simulink model "ADU_Integration_R2014a_simulation"  (R2014a)
settings: Solver=FixedStepDiscrete  StartTime=285  StopTime=300  FixedStep=0.01  RelTol=1e-3
PostLoadFcn:
  | , if any(exist('dsrtsu_mdlpostloadfcn', 'file') == [2, 3, 6]), try dsrtsu_mdlpostloadfcn('Execute', bdroot); catch fprintf('Error in PostLoadFcn (dsrtsu_mdlpostloadfcn) for model "%s":\n %s\n', bdroot, lasterr); end, end,
InitFcn:
  | load 'data/chi2_dat';
  | load 'data/Line_struct';
  | load 'data/innerLNM_1';
  | load 'data/middleLNM_2';
  | load 'data/outerLNM_1';
  | load 'data/landmarks_patac_schimmel_ccw';
  | load 'data/patac_navi_array';
  | load 'data/sensor';
  | load 'data/map_struct';
  | addpath map_src
  | Integration_Parameter;
  | load 'TestData_001';
values from neighbouring files (symbols this model uses):
  TestData_001 =     [TestData_001.mat]
undefined symbols (not defined in the file or in its folder): chi2_dat, innerLNM_1, landmarks_patac_schimmel_ccw, middleLNM_2, outerLNM_1, patac_navi_array
libraries: simulink x36, rtican x1
(part 6 of 22)

== system ADU_Integration_R2014a_simulation/LogData/Sensor_ESR/Data_51 ==
  1-D Lookup Table1 : Lookup_n-D  NumberOfTableDimensions=1  BreakpointsForDimension1=TestData_001.X.Data  Table=TestData_001.Y(206+4*a).Data  RndMeth=Simplest  InputSameDT=on
  1-D Lookup Table2 : Lookup_n-D  NumberOfTableDimensions=1  BreakpointsForDimension1=TestData_001.X.Data  Table=TestData_001.Y(205+4*a).Data  RndMeth=Simplest  InputSameDT=on
  1-D Lookup Table3 : Lookup_n-D  NumberOfTableDimensions=1  BreakpointsForDimension1=TestData_001.X.Data  Table=TestData_001.Y(207+4*a).Data  RndMeth=Simplest  InputSameDT=on
  1-D Lookup Table4 : Lookup_n-D  NumberOfTableDimensions=1  BreakpointsForDimension1=TestData_001.X.Data  Table=TestData_001.Y(208+4*a).Data  RndMeth=Simplest  InputSameDT=on
  Mux5 : Mux
  Quantizer9 : Quantizer  QuantizationInterval=1
  Out1 : Outport
  wires:
  Mux5/1 -> Out1/1
  [Clock] -> 1-D Lookup Table2/1, 1-D Lookup Table4/1, 1-D Lookup Table3/1, 1-D Lookup Table1/1
  1-D Lookup Table4/1 -> Mux5/4
  Quantizer9/1 -> Mux5/1
  1-D Lookup Table2/1 -> Quantizer9/1
  1-D Lookup Table1/1 -> Mux5/2  "Data"
  1-D Lookup Table3/1 -> Mux5/3

== system ADU_Integration_R2014a_simulation/LogData/Sensor_ESR/Data_52 ==
  1-D Lookup Table1 : Lookup_n-D  NumberOfTableDimensions=1  BreakpointsForDimension1=TestData_001.X.Data  Table=TestData_001.Y(206+4*a).Data  RndMeth=Simplest  InputSameDT=on
  1-D Lookup Table2 : Lookup_n-D  NumberOfTableDimensions=1  BreakpointsForDimension1=TestData_001.X.Data  Table=TestData_001.Y(205+4*a).Data  RndMeth=Simplest  InputSameDT=on
  1-D Lookup Table3 : Lookup_n-D  NumberOfTableDimensions=1  BreakpointsForDimension1=TestData_001.X.Data  Table=TestData_001.Y(207+4*a).Data  RndMeth=Simplest  InputSameDT=on
  1-D Lookup Table4 : Lookup_n-D  NumberOfTableDimensions=1  BreakpointsForDimension1=TestData_001.X.Data  Table=TestData_001.Y(208+4*a).Data  RndMeth=Simplest  InputSameDT=on
  Mux5 : Mux
  Quantizer9 : Quantizer  QuantizationInterval=1
  Out1 : Outport
  wires:
  1-D Lookup Table3/1 -> Mux5/3
  1-D Lookup Table1/1 -> Mux5/2  "Data"
  1-D Lookup Table2/1 -> Quantizer9/1
  Quantizer9/1 -> Mux5/1
  1-D Lookup Table4/1 -> Mux5/4
  [Clock] -> 1-D Lookup Table1/1, 1-D Lookup Table3/1, 1-D Lookup Table4/1, 1-D Lookup Table2/1
  Mux5/1 -> Out1/1

== system ADU_Integration_R2014a_simulation/LogData/Sensor_ESR/Data_53 ==
  1-D Lookup Table1 : Lookup_n-D  NumberOfTableDimensions=1  BreakpointsForDimension1=TestData_001.X.Data  Table=TestData_001.Y(206+4*a).Data  RndMeth=Simplest  InputSameDT=on
  1-D Lookup Table2 : Lookup_n-D  NumberOfTableDimensions=1  BreakpointsForDimension1=TestData_001.X.Data  Table=TestData_001.Y(205+4*a).Data  RndMeth=Simplest  InputSameDT=on
  1-D Lookup Table3 : Lookup_n-D  NumberOfTableDimensions=1  BreakpointsForDimension1=TestData_001.X.Data  Table=TestData_001.Y(207+4*a).Data  RndMeth=Simplest  InputSameDT=on
  1-D Lookup Table4 : Lookup_n-D  NumberOfTableDimensions=1  BreakpointsForDimension1=TestData_001.X.Data  Table=TestData_001.Y(208+4*a).Data  RndMeth=Simplest  InputSameDT=on
  Mux5 : Mux
  Quantizer9 : Quantizer  QuantizationInterval=1
  Out1 : Outport
  wires:
  Mux5/1 -> Out1/1
  [Clock] -> 1-D Lookup Table2/1, 1-D Lookup Table4/1, 1-D Lookup Table3/1, 1-D Lookup Table1/1
  1-D Lookup Table4/1 -> Mux5/4
  Quantizer9/1 -> Mux5/1
  1-D Lookup Table2/1 -> Quantizer9/1
  1-D Lookup Table1/1 -> Mux5/2  "Data"
  1-D Lookup Table3/1 -> Mux5/3

== system ADU_Integration_R2014a_simulation/LogData/Sensor_ESR/Data_54 ==
  1-D Lookup Table1 : Lookup_n-D  NumberOfTableDimensions=1  BreakpointsForDimension1=TestData_001.X.Data  Table=TestData_001.Y(206+4*a).Data  RndMeth=Simplest  InputSameDT=on
  1-D Lookup Table2 : Lookup_n-D  NumberOfTableDimensions=1  BreakpointsForDimension1=TestData_001.X.Data  Table=TestData_001.Y(205+4*a).Data  RndMeth=Simplest  InputSameDT=on
  1-D Lookup Table3 : Lookup_n-D  NumberOfTableDimensions=1  BreakpointsForDimension1=TestData_001.X.Data  Table=TestData_001.Y(207+4*a).Data  RndMeth=Simplest  InputSameDT=on
  1-D Lookup Table4 : Lookup_n-D  NumberOfTableDimensions=1  BreakpointsForDimension1=TestData_001.X.Data  Table=TestData_001.Y(208+4*a).Data  RndMeth=Simplest  InputSameDT=on
  Mux5 : Mux
  Quantizer9 : Quantizer  QuantizationInterval=1
  Out1 : Outport
  wires:
  1-D Lookup Table3/1 -> Mux5/3
  1-D Lookup Table1/1 -> Mux5/2  "Data"
  1-D Lookup Table2/1 -> Quantizer9/1
  Quantizer9/1 -> Mux5/1
  1-D Lookup Table4/1 -> Mux5/4
  [Clock] -> 1-D Lookup Table1/1, 1-D Lookup Table3/1, 1-D Lookup Table4/1, 1-D Lookup Table2/1
  Mux5/1 -> Out1/1

== system ADU_Integration_R2014a_simulation/LogData/Sensor_ESR/Data_55 ==
  1-D Lookup Table1 : Lookup_n-D  NumberOfTableDimensions=1  BreakpointsForDimension1=TestData_001.X.Data  Table=TestData_001.Y(206+4*a).Data  RndMeth=Simplest  InputSameDT=on
  1-D Lookup Table2 : Lookup_n-D  NumberOfTableDimensions=1  BreakpointsForDimension1=TestData_001.X.Data  Table=TestData_001.Y(205+4*a).Data  RndMeth=Simplest  InputSameDT=on
  1-D Lookup Table3 : Lookup_n-D  NumberOfTableDimensions=1  BreakpointsForDimension1=TestData_001.X.Data  Table=TestData_001.Y(207+4*a).Data  RndMeth=Simplest  InputSameDT=on
  1-D Lookup Table4 : Lookup_n-D  NumberOfTableDimensions=1  BreakpointsForDimension1=TestData_001.X.Data  Table=TestData_001.Y(208+4*a).Data  RndMeth=Simplest  InputSameDT=on
  Mux5 : Mux
  Quantizer9 : Quantizer  QuantizationInterval=1
  Out1 : Outport
  wires:
  Mux5/1 -> Out1/1
  [Clock] -> 1-D Lookup Table2/1, 1-D Lookup Table4/1, 1-D Lookup Table3/1, 1-D Lookup Table1/1
  1-D Lookup Table4/1 -> Mux5/4
  Quantizer9/1 -> Mux5/1
  1-D Lookup Table2/1 -> Quantizer9/1
  1-D Lookup Table1/1 -> Mux5/2  "Data"
  1-D Lookup Table3/1 -> Mux5/3

== system ADU_Integration_R2014a_simulation/LogData/Sensor_ESR/Data_56 ==
  1-D Lookup Table1 : Lookup_n-D  NumberOfTableDimensions=1  BreakpointsForDimension1=TestData_001.X.Data  Table=TestData_001.Y(206+4*a).Data  RndMeth=Simplest  InputSameDT=on
  1-D Lookup Table2 : Lookup_n-D  NumberOfTableDimensions=1  BreakpointsForDimension1=TestData_001.X.Data  Table=TestData_001.Y(205+4*a).Data  RndMeth=Simplest  InputSameDT=on
  1-D Lookup Table3 : Lookup_n-D  NumberOfTableDimensions=1  BreakpointsForDimension1=TestData_001.X.Data  Table=TestData_001.Y(207+4*a).Data  RndMeth=Simplest  InputSameDT=on
  1-D Lookup Table4 : Lookup_n-D  NumberOfTableDimensions=1  BreakpointsForDimension1=TestData_001.X.Data  Table=TestData_001.Y(208+4*a).Data  RndMeth=Simplest  InputSameDT=on
  Mux5 : Mux
  Quantizer9 : Quantizer  QuantizationInterval=1
  Out1 : Outport
  wires:
  1-D Lookup Table3/1 -> Mux5/3
  1-D Lookup Table1/1 -> Mux5/2  "Data"
  1-D Lookup Table2/1 -> Quantizer9/1
  Quantizer9/1 -> Mux5/1
  1-D Lookup Table4/1 -> Mux5/4
  [Clock] -> 1-D Lookup Table1/1, 1-D Lookup Table3/1, 1-D Lookup Table4/1, 1-D Lookup Table2/1
  Mux5/1 -> Out1/1

== system ADU_Integration_R2014a_simulation/LogData/Sensor_ESR/Data_57 ==
  1-D Lookup Table1 : Lookup_n-D  NumberOfTableDimensions=1  BreakpointsForDimension1=TestData_001.X.Data  Table=TestData_001.Y(206+4*a).Data  RndMeth=Simplest  InputSameDT=on
  1-D Lookup Table2 : Lookup_n-D  NumberOfTableDimensions=1  BreakpointsForDimension1=TestData_001.X.Data  Table=TestData_001.Y(205+4*a).Data  RndMeth=Simplest  InputSameDT=on
  1-D Lookup Table3 : Lookup_n-D  NumberOfTableDimensions=1  BreakpointsForDimension1=TestData_001.X.Data  Table=TestData_001.Y(207+4*a).Data  RndMeth=Simplest  InputSameDT=on
  1-D Lookup Table4 : Lookup_n-D  NumberOfTableDimensions=1  BreakpointsForDimension1=TestData_001.X.Data  Table=TestData_001.Y(208+4*a).Data  RndMeth=Simplest  InputSameDT=on
  Mux5 : Mux
  Quantizer9 : Quantizer  QuantizationInterval=1
  Out1 : Outport
  wires:
  Mux5/1 -> Out1/1
  [Clock] -> 1-D Lookup Table2/1, 1-D Lookup Table4/1, 1-D Lookup Table3/1, 1-D Lookup Table1/1
  1-D Lookup Table4/1 -> Mux5/4
  Quantizer9/1 -> Mux5/1
  1-D Lookup Table2/1 -> Quantizer9/1
  1-D Lookup Table1/1 -> Mux5/2  "Data"
  1-D Lookup Table3/1 -> Mux5/3

== system ADU_Integration_R2014a_simulation/LogData/Sensor_ESR/Data_58 ==
  1-D Lookup Table1 : Lookup_n-D  NumberOfTableDimensions=1  BreakpointsForDimension1=TestData_001.X.Data  Table=TestData_001.Y(206+4*a).Data  RndMeth=Simplest  InputSameDT=on
  1-D Lookup Table2 : Lookup_n-D  NumberOfTableDimensions=1  BreakpointsForDimension1=TestData_001.X.Data  Table=TestData_001.Y(205+4*a).Data  RndMeth=Simplest  InputSameDT=on
  1-D Lookup Table3 : Lookup_n-D  NumberOfTableDimensions=1  BreakpointsForDimension1=TestData_001.X.Data  Table=TestData_001.Y(207+4*a).Data  RndMeth=Simplest  InputSameDT=on
  1-D Lookup Table4 : Lookup_n-D  NumberOfTableDimensions=1  BreakpointsForDimension1=TestData_001.X.Data  Table=TestData_001.Y(208+4*a).Data  RndMeth=Simplest  InputSameDT=on
  Mux5 : Mux
  Quantizer9 : Quantizer  QuantizationInterval=1
  Out1 : Outport
  wires:
  1-D Lookup Table3/1 -> Mux5/3
  1-D Lookup Table1/1 -> Mux5/2  "Data"
  1-D Lookup Table2/1 -> Quantizer9/1
  Quantizer9/1 -> Mux5/1
  1-D Lookup Table4/1 -> Mux5/4
  [Clock] -> 1-D Lookup Table1/1, 1-D Lookup Table3/1, 1-D Lookup Table4/1, 1-D Lookup Table2/1
  Mux5/1 -> Out1/1

== system ADU_Integration_R2014a_simulation/LogData/Sensor_ESR/Data_59 ==
  1-D Lookup Table1 : Lookup_n-D  NumberOfTableDimensions=1  BreakpointsForDimension1=TestData_001.X.Data  Table=TestData_001.Y(206+4*a).Data  RndMeth=Simplest  InputSameDT=on
  1-D Lookup Table2 : Lookup_n-D  NumberOfTableDimensions=1  BreakpointsForDimension1=TestData_001.X.Data  Table=TestData_001.Y(205+4*a).Data  RndMeth=Simplest  InputSameDT=on
  1-D Lookup Table3 : Lookup_n-D  NumberOfTableDimensions=1  BreakpointsForDimension1=TestData_001.X.Data  Table=TestData_001.Y(207+4*a).Data  RndMeth=Simplest  InputSameDT=on
  1-D Lookup Table4 : Lookup_n-D  NumberOfTableDimensions=1  BreakpointsForDimension1=TestData_001.X.Data  Table=TestData_001.Y(208+4*a).Data  RndMeth=Simplest  InputSameDT=on
  Mux5 : Mux
  Quantizer9 : Quantizer  QuantizationInterval=1
  Out1 : Outport
  wires:
  Mux5/1 -> Out1/1
  [Clock] -> 1-D Lookup Table2/1, 1-D Lookup Table4/1, 1-D Lookup Table3/1, 1-D Lookup Table1/1
  1-D Lookup Table4/1 -> Mux5/4
  Quantizer9/1 -> Mux5/1
  1-D Lookup Table2/1 -> Quantizer9/1
  1-D Lookup Table1/1 -> Mux5/2  "Data"
  1-D Lookup Table3/1 -> Mux5/3

== system ADU_Integration_R2014a_simulation/LogData/Sensor_ESR/Data_6 ==
  1-D Lookup Table1 : Lookup_n-D  NumberOfTableDimensions=1  BreakpointsForDimension1=TestData_001.X.Data  Table=TestData_001.Y(206+4*a).Data  RndMeth=Simplest  InputSameDT=on
  1-D Lookup Table2 : Lookup_n-D  NumberOfTableDimensions=1  BreakpointsForDimension1=TestData_001.X.Data  Table=TestData_001.Y(205+4*a).Data  RndMeth=Simplest  InputSameDT=on
  1-D Lookup Table3 : Lookup_n-D  NumberOfTableDimensions=1  BreakpointsForDimension1=TestData_001.X.Data  Table=TestData_001.Y(207+4*a).Data  RndMeth=Simplest  InputSameDT=on
  1-D Lookup Table4 : Lookup_n-D  NumberOfTableDimensions=1  BreakpointsForDimension1=TestData_001.X.Data  Table=TestData_001.Y(208+4*a).Data  RndMeth=Simplest  InputSameDT=on
  Mux5 : Mux
  Quantizer9 : Quantizer  QuantizationInterval=1
  Out1 : Outport
  wires:
  1-D Lookup Table3/1 -> Mux5/3
  1-D Lookup Table1/1 -> Mux5/2  "Data"
  1-D Lookup Table2/1 -> Quantizer9/1
  Quantizer9/1 -> Mux5/1
  1-D Lookup Table4/1 -> Mux5/4
  [Clock] -> 1-D Lookup Table1/1, 1-D Lookup Table3/1, 1-D Lookup Table4/1, 1-D Lookup Table2/1
  Mux5/1 -> Out1/1

== system ADU_Integration_R2014a_simulation/LogData/Sensor_ESR/Data_60 ==
  1-D Lookup Table1 : Lookup_n-D  NumberOfTableDimensions=1  BreakpointsForDimension1=TestData_001.X.Data  Table=TestData_001.Y(206+4*a).Data  RndMeth=Simplest  InputSameDT=on
  1-D Lookup Table2 : Lookup_n-D  NumberOfTableDimensions=1  BreakpointsForDimension1=TestData_001.X.Data  Table=TestData_001.Y(205+4*a).Data  RndMeth=Simplest  InputSameDT=on
  1-D Lookup Table3 : Lookup_n-D  NumberOfTableDimensions=1  BreakpointsForDimension1=TestData_001.X.Data  Table=TestData_001.Y(207+4*a).Data  RndMeth=Simplest  InputSameDT=on
  1-D Lookup Table4 : Lookup_n-D  NumberOfTableDimensions=1  BreakpointsForDimension1=TestData_001.X.Data  Table=TestData_001.Y(208+4*a).Data  RndMeth=Simplest  InputSameDT=on
  Mux5 : Mux
  Quantizer9 : Quantizer  QuantizationInterval=1
  Out1 : Outport
  wires:
  1-D Lookup Table3/1 -> Mux5/3
  1-D Lookup Table1/1 -> Mux5/2  "Data"
  1-D Lookup Table2/1 -> Quantizer9/1
  Quantizer9/1 -> Mux5/1
  1-D Lookup Table4/1 -> Mux5/4
  [Clock] -> 1-D Lookup Table1/1, 1-D Lookup Table3/1, 1-D Lookup Table4/1, 1-D Lookup Table2/1
  Mux5/1 -> Out1/1

== system ADU_Integration_R2014a_simulation/LogData/Sensor_ESR/Data_61 ==
  1-D Lookup Table1 : Lookup_n-D  NumberOfTableDimensions=1  BreakpointsForDimension1=TestData_001.X.Data  Table=TestData_001.Y(206+4*a).Data  RndMeth=Simplest  InputSameDT=on
  1-D Lookup Table2 : Lookup_n-D  NumberOfTableDimensions=1  BreakpointsForDimension1=TestData_001.X.Data  Table=TestData_001.Y(205+4*a).Data  RndMeth=Simplest  InputSameDT=on
  1-D Lookup Table3 : Lookup_n-D  NumberOfTableDimensions=1  BreakpointsForDimension1=TestData_001.X.Data  Table=TestData_001.Y(207+4*a).Data  RndMeth=Simplest  InputSameDT=on
  1-D Lookup Table4 : Lookup_n-D  NumberOfTableDimensions=1  BreakpointsForDimension1=TestData_001.X.Data  Table=TestData_001.Y(208+4*a).Data  RndMeth=Simplest  InputSameDT=on
  Mux5 : Mux
  Quantizer9 : Quantizer  QuantizationInterval=1
  Out1 : Outport
  wires:
  Mux5/1 -> Out1/1
  [Clock] -> 1-D Lookup Table2/1, 1-D Lookup Table4/1, 1-D Lookup Table3/1, 1-D Lookup Table1/1
  1-D Lookup Table4/1 -> Mux5/4
  Quantizer9/1 -> Mux5/1
  1-D Lookup Table2/1 -> Quantizer9/1
  1-D Lookup Table1/1 -> Mux5/2  "Data"
  1-D Lookup Table3/1 -> Mux5/3

== system ADU_Integration_R2014a_simulation/LogData/Sensor_ESR/Data_62 ==
  1-D Lookup Table1 : Lookup_n-D  NumberOfTableDimensions=1  BreakpointsForDimension1=TestData_001.X.Data  Table=TestData_001.Y(206+4*a).Data  RndMeth=Simplest  InputSameDT=on
  1-D Lookup Table2 : Lookup_n-D  NumberOfTableDimensions=1  BreakpointsForDimension1=TestData_001.X.Data  Table=TestData_001.Y(205+4*a).Data  RndMeth=Simplest  InputSameDT=on
  1-D Lookup Table3 : Lookup_n-D  NumberOfTableDimensions=1  BreakpointsForDimension1=TestData_001.X.Data  Table=TestData_001.Y(207+4*a).Data  RndMeth=Simplest  InputSameDT=on
  1-D Lookup Table4 : Lookup_n-D  NumberOfTableDimensions=1  BreakpointsForDimension1=TestData_001.X.Data  Table=TestData_001.Y(208+4*a).Data  RndMeth=Simplest  InputSameDT=on
  Mux5 : Mux
  Quantizer9 : Quantizer  QuantizationInterval=1
  Out1 : Outport
  wires:
  1-D Lookup Table3/1 -> Mux5/3
  1-D Lookup Table1/1 -> Mux5/2  "Data"
  1-D Lookup Table2/1 -> Quantizer9/1
  Quantizer9/1 -> Mux5/1
  1-D Lookup Table4/1 -> Mux5/4
  [Clock] -> 1-D Lookup Table1/1, 1-D Lookup Table3/1, 1-D Lookup Table4/1, 1-D Lookup Table2/1
  Mux5/1 -> Out1/1

== system ADU_Integration_R2014a_simulation/LogData/Sensor_ESR/Data_63 ==
  1-D Lookup Table1 : Lookup_n-D  NumberOfTableDimensions=1  BreakpointsForDimension1=TestData_001.X.Data  Table=TestData_001.Y(206+4*a).Data  RndMeth=Simplest  InputSameDT=on
  1-D Lookup Table2 : Lookup_n-D  NumberOfTableDimensions=1  BreakpointsForDimension1=TestData_001.X.Data  Table=TestData_001.Y(205+4*a).Data  RndMeth=Simplest  InputSameDT=on
  1-D Lookup Table3 : Lookup_n-D  NumberOfTableDimensions=1  BreakpointsForDimension1=TestData_001.X.Data  Table=TestData_001.Y(207+4*a).Data  RndMeth=Simplest  InputSameDT=on
  1-D Lookup Table4 : Lookup_n-D  NumberOfTableDimensions=1  BreakpointsForDimension1=TestData_001.X.Data  Table=TestData_001.Y(208+4*a).Data  RndMeth=Simplest  InputSameDT=on
  Mux5 : Mux
  Quantizer9 : Quantizer  QuantizationInterval=1
  Out1 : Outport
  wires:
  Mux5/1 -> Out1/1
  [Clock] -> 1-D Lookup Table2/1, 1-D Lookup Table4/1, 1-D Lookup Table3/1, 1-D Lookup Table1/1
  1-D Lookup Table4/1 -> Mux5/4
  Quantizer9/1 -> Mux5/1
  1-D Lookup Table2/1 -> Quantizer9/1
  1-D Lookup Table1/1 -> Mux5/2  "Data"
  1-D Lookup Table3/1 -> Mux5/3

== system ADU_Integration_R2014a_simulation/LogData/Sensor_ESR/Data_64 ==
  1-D Lookup Table1 : Lookup_n-D  NumberOfTableDimensions=1  BreakpointsForDimension1=TestData_001.X.Data  Table=TestData_001.Y(206+4*a).Data  RndMeth=Simplest  InputSameDT=on
  1-D Lookup Table2 : Lookup_n-D  NumberOfTableDimensions=1  BreakpointsForDimension1=TestData_001.X.Data  Table=TestData_001.Y(205+4*a).Data  RndMeth=Simplest  InputSameDT=on
  1-D Lookup Table3 : Lookup_n-D  NumberOfTableDimensions=1  BreakpointsForDimension1=TestData_001.X.Data  Table=TestData_001.Y(207+4*a).Data  RndMeth=Simplest  InputSameDT=on
  1-D Lookup Table4 : Lookup_n-D  NumberOfTableDimensions=1  BreakpointsForDimension1=TestData_001.X.Data  Table=TestData_001.Y(208+4*a).Data  RndMeth=Simplest  InputSameDT=on
  Mux5 : Mux
  Quantizer9 : Quantizer  QuantizationInterval=1
  Out1 : Outport
  wires:
  1-D Lookup Table3/1 -> Mux5/3
  1-D Lookup Table1/1 -> Mux5/2  "Data"
  1-D Lookup Table2/1 -> Quantizer9/1
  Quantizer9/1 -> Mux5/1
  1-D Lookup Table4/1 -> Mux5/4
  [Clock] -> 1-D Lookup Table1/1, 1-D Lookup Table3/1, 1-D Lookup Table4/1, 1-D Lookup Table2/1
  Mux5/1 -> Out1/1

== system ADU_Integration_R2014a_simulation/LogData/Sensor_ESR/Data_7 ==
  1-D Lookup Table1 : Lookup_n-D  NumberOfTableDimensions=1  BreakpointsForDimension1=TestData_001.X.Data  Table=TestData_001.Y(206+4*a).Data  RndMeth=Simplest  InputSameDT=on
  1-D Lookup Table2 : Lookup_n-D  NumberOfTableDimensions=1  BreakpointsForDimension1=TestData_001.X.Data  Table=TestData_001.Y(205+4*a).Data  RndMeth=Simplest  InputSameDT=on
  1-D Lookup Table3 : Lookup_n-D  NumberOfTableDimensions=1  BreakpointsForDimension1=TestData_001.X.Data  Table=TestData_001.Y(207+4*a).Data  RndMeth=Simplest  InputSameDT=on
  1-D Lookup Table4 : Lookup_n-D  NumberOfTableDimensions=1  BreakpointsForDimension1=TestData_001.X.Data  Table=TestData_001.Y(208+4*a).Data  RndMeth=Simplest  InputSameDT=on
  Mux5 : Mux
  Quantizer9 : Quantizer  QuantizationInterval=1
  Out1 : Outport
  wires:
  Mux5/1 -> Out1/1
  [Clock] -> 1-D Lookup Table2/1, 1-D Lookup Table4/1, 1-D Lookup Table3/1, 1-D Lookup Table1/1
  1-D Lookup Table4/1 -> Mux5/4
  Quantizer9/1 -> Mux5/1
  1-D Lookup Table2/1 -> Quantizer9/1
  1-D Lookup Table1/1 -> Mux5/2  "Data"
  1-D Lookup Table3/1 -> Mux5/3

== system ADU_Integration_R2014a_simulation/LogData/Sensor_ESR/Data_8 ==
  1-D Lookup Table1 : Lookup_n-D  NumberOfTableDimensions=1  BreakpointsForDimension1=TestData_001.X.Data  Table=TestData_001.Y(206+4*a).Data  RndMeth=Simplest  InputSameDT=on
  1-D Lookup Table2 : Lookup_n-D  NumberOfTableDimensions=1  BreakpointsForDimension1=TestData_001.X.Data  Table=TestData_001.Y(205+4*a).Data  RndMeth=Simplest  InputSameDT=on
  1-D Lookup Table3 : Lookup_n-D  NumberOfTableDimensions=1  BreakpointsForDimension1=TestData_001.X.Data  Table=TestData_001.Y(207+4*a).Data  RndMeth=Simplest  InputSameDT=on
  1-D Lookup Table4 : Lookup_n-D  NumberOfTableDimensions=1  BreakpointsForDimension1=TestData_001.X.Data  Table=TestData_001.Y(208+4*a).Data  RndMeth=Simplest  InputSameDT=on
  Mux5 : Mux
  Quantizer9 : Quantizer  QuantizationInterval=1
  Out1 : Outport
  wires:
  1-D Lookup Table3/1 -> Mux5/3
  1-D Lookup Table1/1 -> Mux5/2  "Data"
  1-D Lookup Table2/1 -> Quantizer9/1
  Quantizer9/1 -> Mux5/1
  1-D Lookup Table4/1 -> Mux5/4
  [Clock] -> 1-D Lookup Table1/1, 1-D Lookup Table3/1, 1-D Lookup Table4/1, 1-D Lookup Table2/1
  Mux5/1 -> Out1/1

== system ADU_Integration_R2014a_simulation/LogData/Sensor_ESR/Data_9 ==
  1-D Lookup Table1 : Lookup_n-D  NumberOfTableDimensions=1  BreakpointsForDimension1=TestData_001.X.Data  Table=TestData_001.Y(206+4*a).Data  RndMeth=Simplest  InputSameDT=on
  1-D Lookup Table2 : Lookup_n-D  NumberOfTableDimensions=1  BreakpointsForDimension1=TestData_001.X.Data  Table=TestData_001.Y(205+4*a).Data  RndMeth=Simplest  InputSameDT=on
  1-D Lookup Table3 : Lookup_n-D  NumberOfTableDimensions=1  BreakpointsForDimension1=TestData_001.X.Data  Table=TestData_001.Y(207+4*a).Data  RndMeth=Simplest  InputSameDT=on
  1-D Lookup Table4 : Lookup_n-D  NumberOfTableDimensions=1  BreakpointsForDimension1=TestData_001.X.Data  Table=TestData_001.Y(208+4*a).Data  RndMeth=Simplest  InputSameDT=on
  Mux5 : Mux
  Quantizer9 : Quantizer  QuantizationInterval=1
  Out1 : Outport
  wires:
  Mux5/1 -> Out1/1
  [Clock] -> 1-D Lookup Table2/1, 1-D Lookup Table4/1, 1-D Lookup Table3/1, 1-D Lookup Table1/1
  1-D Lookup Table4/1 -> Mux5/4
  Quantizer9/1 -> Mux5/1
  1-D Lookup Table2/1 -> Quantizer9/1
  1-D Lookup Table1/1 -> Mux5/2  "Data"
  1-D Lookup Table3/1 -> Mux5/3
